simulink model "Cubesat_Control_System"  (R2025b)
settings: Solver=ode45  StartTime=0.0  StopTime=t_stop  RelTol=1e-3
values from neighbouring files (symbols this model uses):
  J = 0.002    [init_simulation.m]    (also in init_simulation_lqr.m)
  Jw = 1e-5    (= 1e-05)    [init_simulation.m]    (also in init_simulation_lqr.m)
  Kd = 0.01    [init_simulation.m]
  Kd_detumble = 0.03    [init_simulation.m]    (also in init_simulation_lqr.m = lqr(A_d, B_d, Q_d, R_d))
  Kp = 0.02    [init_simulation.m]
  omega0 = deg2rad(omega0_deg)    [init_simulation.m]    (also in init_simulation_lqr.m)
  omega_th_high = deg2rad(10000)    [init_simulation.m]    (also in init_simulation_lqr.m)
  omega_th_low = deg2rad(0.3)    [init_simulation.m]    (also in init_simulation_lqr.m)
  omega_w0 = 0    [init_simulation.m]    (also in init_simulation_lqr.m)
  tau_max = 0.002    [init_simulation.m]    (also in init_simulation_lqr.m)
  theta0 = deg2rad(0)    [init_simulation.m]    (also in init_simulation_lqr.m)
  theta_ref = deg2rad(theta_ref_deg)    [init_simulation.m]    (also in init_simulation_lqr.m)
settings Model: Creator=bbtp  LastModifiedBy=bbtp

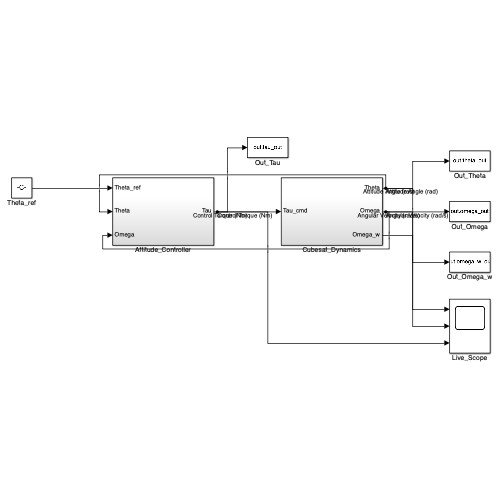
[thumbnail: Simulink's stored preview of the top-level diagram]
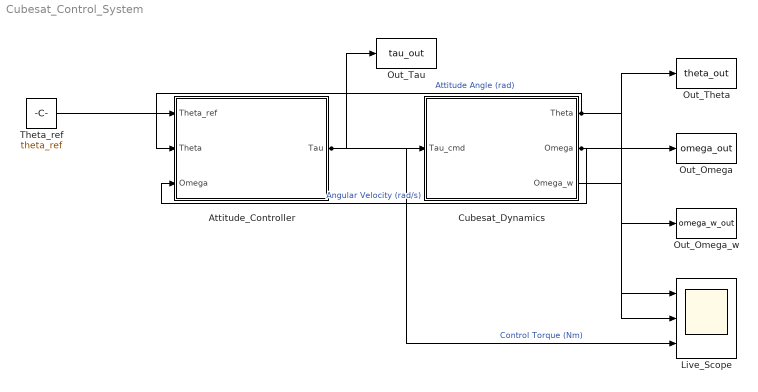
== system Cubesat_Control_System ==
  Attitude_Controller : Subsystem
  Cubesat_Dynamics : Subsystem
  Live_Scope : Scope  NumInputPorts=3
  Out_Omega : ToWorkspace  VariableName=omega_out  SampleTime=-1
  Out_Omega_w : ToWorkspace  VariableName=omega_w_out  SampleTime=-1
  Out_Tau : ToWorkspace  VariableName=tau_out  SampleTime=-1
  Out_Theta : ToWorkspace  VariableName=theta_out  SampleTime=-1
  Theta_ref : Constant  Value=theta_ref
  wires:
  Theta_ref/1 -> Attitude_Controller/1(Theta_ref)
  Attitude_Controller/1(Tau) -> Cubesat_Dynamics/1(Tau_cmd), Out_Tau/1, Live_Scope/3  "Control Torque (Nm)"
  Cubesat_Dynamics/1(Theta) -> Out_Theta/1, Attitude_Controller/2(Theta), Live_Scope/1  "Attitude Angle (rad)"
  Cubesat_Dynamics/2(Omega) -> Out_Omega/1, Attitude_Controller/3(Omega), Live_Scope/2  "Angular Velocity (rad/s)"
  Cubesat_Dynamics/3(Omega_w) -> Out_Omega_w/1

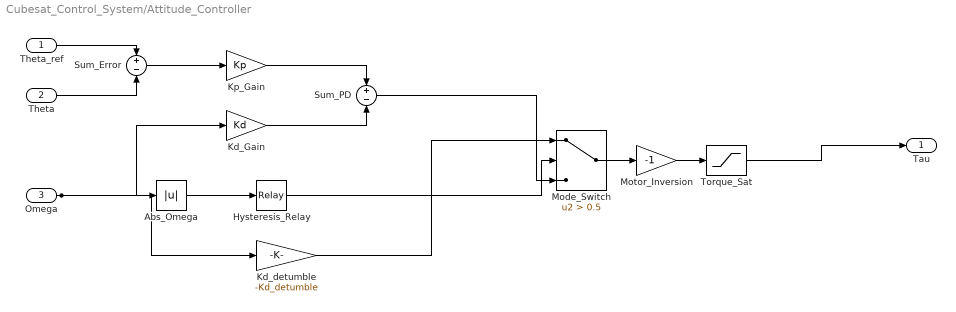
== system Cubesat_Control_System/Attitude_Controller ==
  Theta_ref : Inport
  Theta : Inport  Port=2
  Omega : Inport  Port=3
  Abs_Omega : Abs  SaturateOnIntegerOverflow=off
  Hysteresis_Relay : Relay  OnSwitchValue=omega_th_high  OffSwitchValue=omega_th_low
  Kd_Gain : Gain  Gain=Kd
  Kd_detumble : Gain  Gain=-Kd_detumble
  Kp_Gain : Gain  Gain=Kp
  Mode_Switch : Switch  Criteria=u2 > Threshold  Threshold=0.5  SaturateOnIntegerOverflow=off  InputSameDT=off
  Motor_Inversion : Gain  Gain=-1
  Sum_Error : Sum  Inputs=+-
  Sum_PD : Sum  Inputs=+-
  Torque_Sat : Saturate  UpperLimit=tau_max  LowerLimit=-tau_max
  Tau : Outport
  wires:
  ? -> ?
  Theta_ref/1 -> Sum_Error/1
  Theta/1 -> Sum_Error/2
  Sum_Error/1 -> Kp_Gain/1
  Omega/1 -> Kd_Gain/1, Kd_detumble/1, Abs_Omega/1
  Kp_Gain/1 -> Sum_PD/1
  Kd_Gain/1 -> Sum_PD/2
  Kd_detumble/1 -> Mode_Switch/1
  Abs_Omega/1 -> Hysteresis_Relay/1
  Hysteresis_Relay/1 -> Mode_Switch/2
  Sum_PD/1 -> Mode_Switch/3
  Mode_Switch/1 -> Motor_Inversion/1
  Motor_Inversion/1 -> Torque_Sat/1
  Torque_Sat/1 -> Tau/1

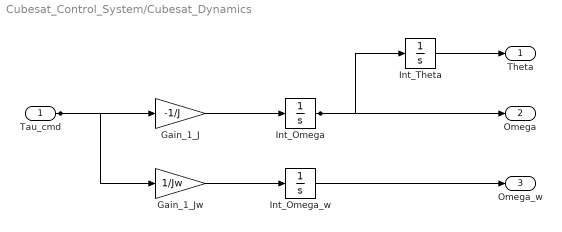
== system Cubesat_Control_System/Cubesat_Dynamics ==
  Tau_cmd : Inport
  Gain_1_J : Gain  Gain=-1/J
  Gain_1_Jw : Gain  Gain=1/Jw
  Int_Omega : Integrator  InitialCondition=omega0
  Int_Omega_w : Integrator  InitialCondition=omega_w0
  Int_Theta : Integrator  InitialCondition=theta0
  Theta : Outport
  Omega : Outport  Port=2
  Omega_w : Outport  Port=3
  wires:
  ? -> ?
  Tau_cmd/1 -> Gain_1_Jw/1, Gain_1_J/1
  Gain_1_Jw/1 -> Int_Omega_w/1
  Gain_1_J/1 -> Int_Omega/1
  Int_Omega/1 -> Int_Theta/1, Omega/1
  Int_Theta/1 -> Theta/1
  Int_Omega_w/1 -> Omega_w/1
